simulink model "Practica_1"  (R2016a)
settings: Solver=VariableStepAuto  StartTime=0.0  StopTime=10.0  RelTol=1e-3
settings Model: Creator=irvin  LastModifiedBy=irvin

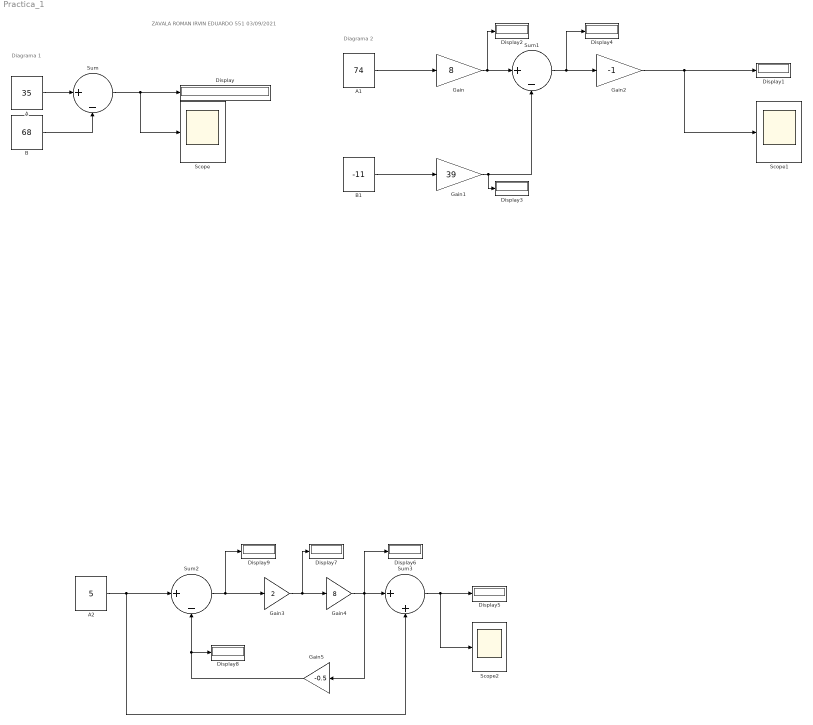
== system Practica_1 ==
  note: ZAVALA ROMAN IRVIN EDUARDO 551 03/09/2021
  note: Diagrama 2
  note: Diagrama 1
  A : Constant  Value=35
  A1 : Constant  Value=74
  A2 : Constant  Value=5
  B : Constant  Value=68
  B1 : Constant  Value=-11
  Display{,1..9} (10 alike) : Display
  Gain : Gain  Gain=8
  Gain1 : Gain  Gain=39
  Gain2 : Gain  Gain=-1
  Gain3 : Gain  Gain=2
  Gain4 : Gain  Gain=8
  Gain5 : Gain  Gain=-0.5
  Scope : Scope
  Scope1 : Scope
  Scope2 : Scope
  Sum : Sum  Inputs=|+-
  Sum1 : Sum  Inputs=|+-
  Sum2 : Sum  Inputs=|+-
  Sum3 : Sum  Inputs=|++
  wires:
  A/1 -> Sum/1
  B/1 -> Sum/2
  Sum/1 -> Scope/1, Display/1
  B1/1 -> Gain1/1
  A1/1 -> Gain/1
  Gain/1 -> Display2/1, Sum1/1
  Gain1/1 -> Display3/1, Sum1/2
  Sum1/1 -> Display4/1, Gain2/1
  Gain2/1 -> Scope1/1, Display1/1
  A2/1 -> Sum3/2, Sum2/1
  Gain3/1 -> Display7/1, Gain4/1
  Sum2/1 -> Display9/1, Gain3/1
  Gain5/1 -> Display8/1, Sum2/2
  Gain4/1 -> Gain5/1, Display6/1, Sum3/1
  Sum3/1 -> Scope2/1, Display5/1
